simulink model "model"  (R2022a)
settings: Solver=VariableStepAuto  StartTime=0.0  StopTime=16000  RelTol=1e-3
values from neighbouring files (symbols this model uses):
  C_index = 3    [parameters.m]    (also in parameters.mat)
  C_r = 6.6    [parameters.m]    (also in parameters.mat)
  Cap_det = -1e-7    (= -1e-07)    [parameters.m]    (also in parameters.mat)
  cCap = awgn(cCap, -60)    [parameters.m]    (also in parameters.mat = [24858.4246179 23482.1280672 24461.5414582 21708.1837001 234)
  cell_count = 126    [parameters.m]    (also in parameters.mat)
  cQur = cCap / 2    [parameters.m]    (also in parameters.mat = [11880 11880 11880 11880 11880 11880 11880 11880 11880 11880)
  cTmp = 20*ones(60, 1)    [parameters.m]    (also in parameters.mat = [20 20 20 20 20 20 20 20 20 20 20 20 ... (60 elements, 60x1))
  I_CV = 1    [parameters.m]    (also in parameters.mat)
  ocv = ocv_LUT    [parameters.m]    (also in parameters.mat = [0 2.99808472822 3.29015678206 3.51449858493 3.66802196423 3)
  Q_index = 2    [parameters.m]    (also in parameters.mat)
  R_short = 33    [parameters.m]    (also in parameters.mat)
  Rp = Rp_LUT    [parameters.m]    (also in parameters.mat = [0.0013284973182 0.00132849731829 0.00133071540687 0.0013310)
  Rs = Rs_LUT    [parameters.m]    (also in parameters.mat = [0.0044622496006 0.00446224960062 0.00395928973129 0.0036572)
  soc = soc_LUT    [parameters.m]    (also in parameters.mat = [0 0.01 0.0909090909091 0.181818181818 0.272727272727 0.3636)
  tau = tau_LUT    [parameters.m]    (also in parameters.mat = [950.87194683 950.871946837 952.459545918 952.715608142 956.)
  Ts = 0.2    [parameters.m]    (also in parameters.mat)
  U_CC = 0.06    [parameters.m]    (also in parameters.mat)
  U_sought = 4.15    [parameters.m]    (also in parameters.mat)
  U_tol = 0.0000005    (= 5e-07)    [parameters.m]    (also in parameters.mat)
undefined symbols (not defined in the file or in its folder): CC_level, CC_true, CV_level, CV_true, Ts_sim
libraries: simulink x3, sharedTrackingLibrary x1, simulink_extras x1
settings Model: Creator=oscar  LastModifiedBy=oscar
settings OptimizationCC: StrengthReduction=on  PassReuseOutputArgsAs=Individual arguments  ZeroExternalMemoryAtStartup=off  ZeroInternalMemoryAtStartup=off  OptimizeBlockOrder=speed  OptimizationPriority=Speed  OptimizationCustomize=off  MultiThreadedLoops=on  EfficientTunableParamExpr=on
settings DebuggingCC: ParameterTunabilityLossMsg=error  UnconnectedInputMsg=warning  UnconnectedOutputMsg=warning  UnconnectedLineMsg=warning
settings HardwareCC: ProdBitPerPointer=32  ProdBitPerSizeT=32  ProdBitPerPtrDiffT=32  ProdLargestAtomicInteger=Long  ProdLargestAtomicFloat=Double  ProdWordSize=32  ProdHWDeviceType=ARM Compatible->ARM Cortex-M
settings SFSimCC: MATLABDynamicMemAlloc=off
settings RTWCC: SystemTargetFile=ert.tlc  GenCodeOnly=on  TemplateMakefile=ert_default_tmf  GenerateReport=on  LaunchReport=on  CodeExecutionProfiling=on  DLArmComputeVersion=19.05
settings CodeAppCC: ForceParamTrailComments=on  GenerateComments=off  IgnoreCustomStorageClasses=off  OperatorAnnotations=on  SimulinkDataObjDesc=on  SFDataObjDesc=on  InsertBlockDesc=on
settings ERTTargetCC: TargetLangStandard=C99 (ISO)  CodeReplacementLibrary=ARM Cortex-M  UtilityFuncGeneration=Shared location  GenerateSampleERTMain=on  SupportComplex=off  ERTCustomFileTemplate=example_file_process.tlc

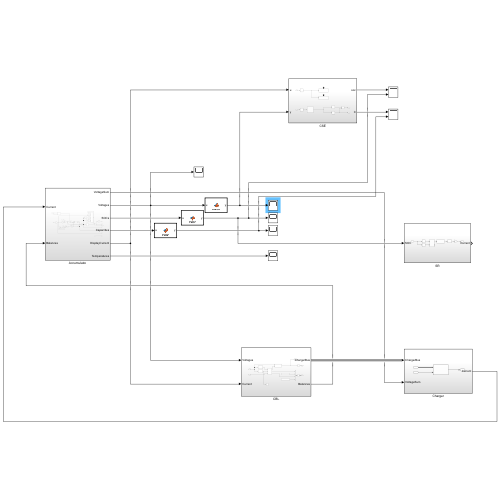
[thumbnail: Simulink's stored preview of the top-level diagram]
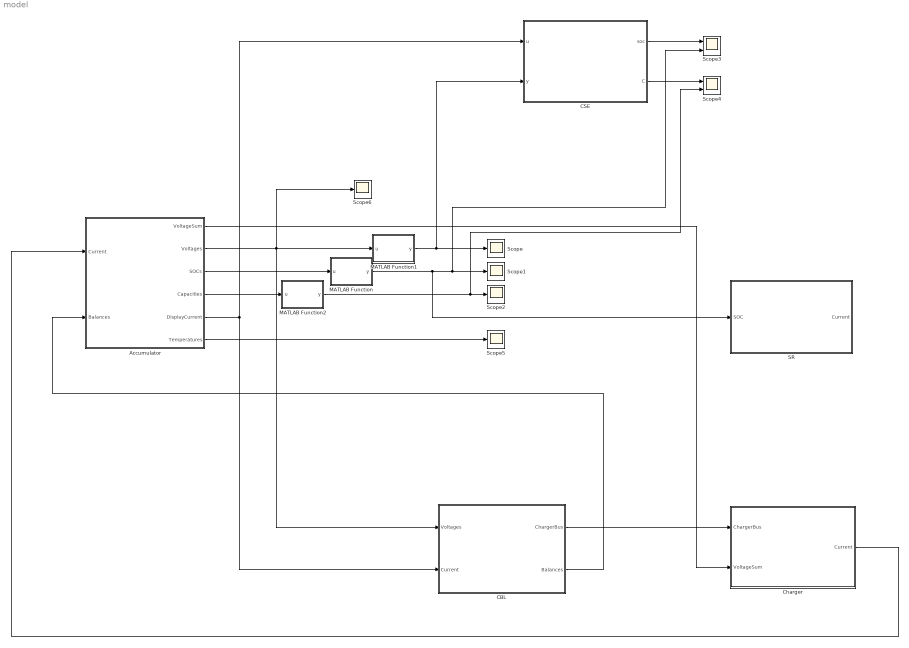
== system model ==
  Accumulator : Subsystem
  CBL : Subsystem
  CSE : Subsystem
  Charger : Subsystem
  MATLAB Function : MATLAB Function  TreatAsAtomicUnit=on
  MATLAB Function1 : MATLAB Function  TreatAsAtomicUnit=on
  MATLAB Function2 : MATLAB Function  TreatAsAtomicUnit=on
  SR : Subsystem
  Scope{,1..2,5..6} (5 alike) : Scope
  Scope3 : Scope  NumInputPorts=2
  Scope4 : Scope  NumInputPorts=2
  wires:
  Accumulator/3(SOCs) -> MATLAB Function/1(u)
  MATLAB Function/1(y) -> Scope1/1, Scope3/2, SR/1(SOC)
  Accumulator/2(Voltages) -> Scope6/1, MATLAB Function1/1(u), CBL/1(Voltages)
  MATLAB Function1/1(y) -> CSE/2(y), Scope/1
  MATLAB Function2/1(y) -> Scope4/2, Scope2/1
  Accumulator/4(Capacities) -> MATLAB Function2/1(u)
  CBL/2(Balances) -> Accumulator/2(Balances)
  CSE/1(soc) -> Scope3/1
  CSE/2(C) -> Scope4/1
  CBL/1(ChargerBus) -> Charger/1(ChargerBus)
  Accumulator/5(DisplayCurrent) -> CBL/2(Current), CSE/1(u)
  Accumulator/6(Temperatures) -> Scope5/1
  Accumulator/1(VoltageSum) -> Charger/2(VoltageSum)
  Charger/1(Current) -> Accumulator/1(Current)

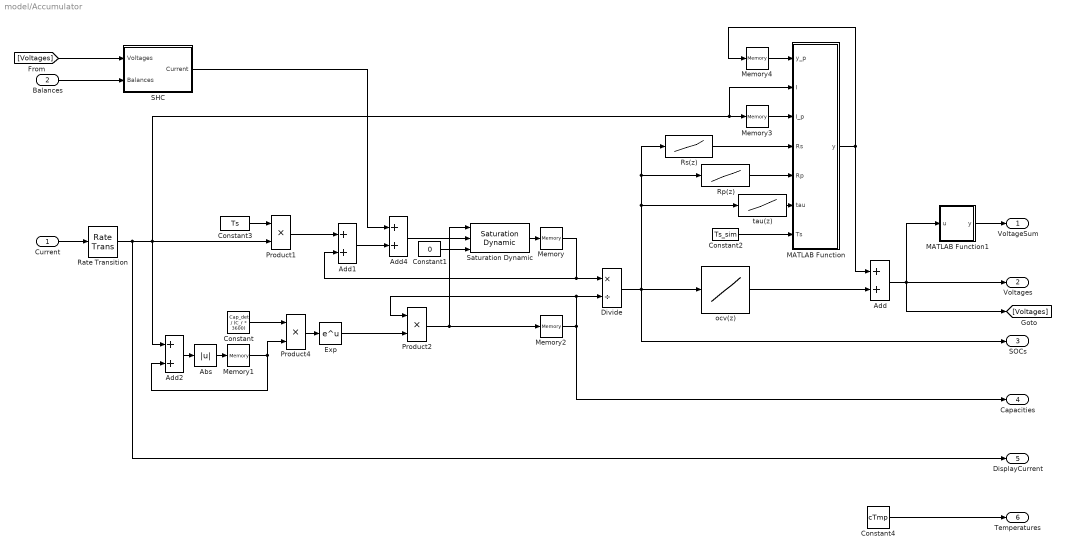
== system model/Accumulator ==
  Current : Inport
  Balances : Inport  Port=2
  Abs : Abs  SaturateOnIntegerOverflow=off
  Add{,1..2,4} (4 alike) : Sum
  Constant : Constant  Value=Cap_det / (C_r * 3600)
  Constant1 : Constant  Value=0
  Constant2 : Constant  Value=Ts_sim
  Constant3 : Constant  Value=Ts
  Constant4 : Constant  Value=cTmp
  Divide : Product  Inputs=*/
  Exp : Math
  MATLAB Function : MATLAB Function  TreatAsAtomicUnit=on
  MATLAB Function1 : MATLAB Function  TreatAsAtomicUnit=on
  Memory : Memory  InitialCondition=cQur
  Memory1 : Memory
  Memory2 : Memory  InitialCondition=cCap
  Memory3 : Memory
  Memory4 : Memory  InitialCondition=zeros(cell_count, 1)
  Product1 : Product
  Product2 : Product
  Product4 : Product
  Rate Transition : RateTransition  OutPortSampleTime=Ts
  Rp(z) : Lookup_n-D  NumberOfTableDimensions=1  BreakpointsForDimension1=soc  Table=Rp  InternalRulePriority=Speed  RndMeth=Simplest
  Rs(z) : Lookup_n-D  NumberOfTableDimensions=1  BreakpointsForDimension1=soc  Table=Rs  InternalRulePriority=Speed  RndMeth=Simplest
  SHC : Subsystem
  Saturation Dynamic : simulink/Discontinuities/Saturation Dynamic  OutMin=[]  OutMax=[]  OutDataTypeStr=Inherit: Same as second input  OutDataType=fixdt(1, 16)  OutScaling=2^-10  DoSatur=off
  ocv(z) : Lookup_n-D  NumberOfTableDimensions=1  BreakpointsForDimension1=soc  Table=ocv  InternalRulePriority=Speed  RndMeth=Simplest
  tau(z) : Lookup_n-D  NumberOfTableDimensions=1  BreakpointsForDimension1=soc  Table=tau  InternalRulePriority=Speed  RndMeth=Simplest
  VoltageSum : Outport
  Voltages : Outport  Port=2
  SOCs : Outport  Port=3
  Capacities : Outport  Port=4
  DisplayCurrent : Outport  Port=5
  Temperatures : Outport  Port=6
  wires:
  Constant/1 -> Product4/1
  Exp/1 -> Product2/2
  Product2/1 -> Saturation Dynamic/1, Memory2/1
  Memory1/1 -> Product4/2, Add2/2
  Abs/1 -> Memory1/1
  Memory/1 -> Divide/1, Add1/2
  Product4/1 -> Exp/1
  Add2/1 -> Abs/1
  Add/1 -> Voltages/1, [Voltages], MATLAB Function1/1(u)
  Saturation Dynamic/1 -> Memory/1
  Constant1/1 -> Saturation Dynamic/3
  Memory3/1 -> MATLAB Function/3(I_p)
  tau(z)/1 -> MATLAB Function/6(tau)
  Rs(z)/1 -> MATLAB Function/4(Rs)
  Rp(z)/1 -> MATLAB Function/5(Rp)
  Memory4/1 -> MATLAB Function/1(y_p)
  MATLAB Function/1(y) -> Memory4/1, Add/1
  Constant2/1 -> MATLAB Function/7(Ts)
  Current/1 -> Rate Transition/1
  Divide/1 -> ocv(z)/1, SOCs/1, tau(z)/1, Rp(z)/1, Rs(z)/1
  Memory2/1 -> Divide/2, Product2/1, Capacities/1
  ocv(z)/1 -> Add/2
  SHC/1(Current) -> Add4/1
  Balances/1 -> SHC/2(Balances)
  Add4/1 -> Saturation Dynamic/2
  [Voltages] -> SHC/1(Voltages)
  Add1/1 -> Add4/2
  Constant4/1 -> Temperatures/1
  Constant3/1 -> Product1/1
  Rate Transition/1 -> Add2/1, Product1/2, MATLAB Function/2(I), Memory3/1, DisplayCurrent/1
  Product1/1 -> Add1/1
  MATLAB Function1/1(y) -> VoltageSum/1

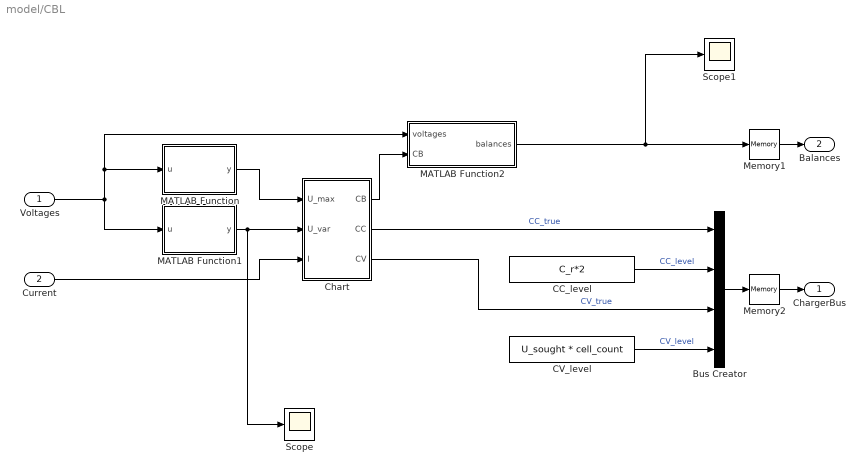
== system model/CBL ==
  Voltages : Inport
  Current : Inport  Port=2
  Bus Creator : BusCreator  Inputs=CC_true,CC_level,CV_true,CV_level
  CC_level : Constant  Value=C_r*2
  CV_level : Constant  Value=U_sought * cell_count
  Chart : Stateflow chart  TreatAsAtomicUnit=on
  MATLAB Function : MATLAB Function  TreatAsAtomicUnit=on
  MATLAB Function1 : MATLAB Function  TreatAsAtomicUnit=on
  MATLAB Function2 : MATLAB Function  TreatAsAtomicUnit=on
  Memory1 : Memory
  Memory2 : Memory
  Scope : Scope
  Scope1 : Scope
  ChargerBus : Outport
  Balances : Outport  Port=2
  wires:
  MATLAB Function/1(y) -> Chart/1(U_max)
  MATLAB Function1/1(y) -> Chart/2(U_var), Scope/1
  Voltages/1 -> MATLAB Function2/1(voltages), MATLAB Function/1(u), MATLAB Function1/1(u)
  Chart/1(CB) -> MATLAB Function2/2(CB)
  MATLAB Function2/1(balances) -> Scope1/1, Memory1/1
  Memory1/1 -> Balances/1
  Bus Creator/1 -> Memory2/1
  Current/1 -> Chart/3(I)
  CC_level/1 -> Bus Creator/2  "CC_level"
  Chart/2(CC) -> Bus Creator/1  "CC_true"
  Chart/3(CV) -> Bus Creator/3  "CV_true"
  CV_level/1 -> Bus Creator/4  "CV_level"
  Memory2/1 -> ChargerBus/1

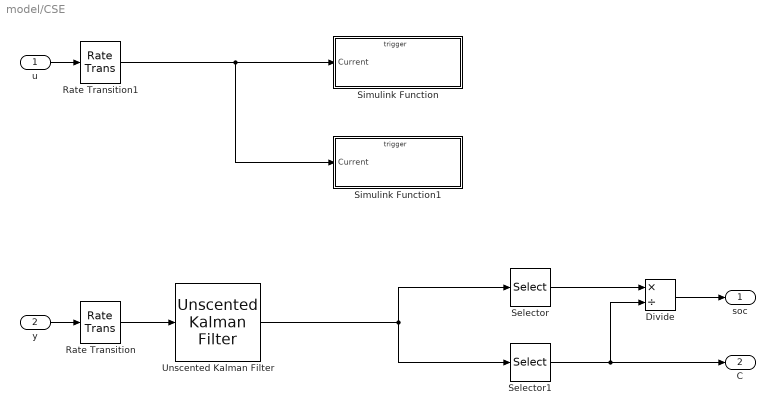
== system model/CSE ==
  u : Inport
  y : Inport  Port=2
  Divide : Product  Inputs=*/
  Rate Transition : RateTransition  OutPortSampleTime=Ts
  Rate Transition1 : RateTransition  OutPortSampleTime=Ts
  Selector : Selector  InputPortWidth=l_x  IndexOptions=Index vector (dialog)  Indices=[Q_index]  OutputSizes=1
  Selector1 : Selector  InputPortWidth=l_x  IndexOptions=Index vector (dialog)  Indices=[C_index]  OutputSizes=1
  Simulink Function : Subsystem  TreatAsAtomicUnit=on
  Simulink Function1 : Subsystem  TreatAsAtomicUnit=on
  Unscented Kalman Filter : sharedTrackingLibrary/Unscented Kalman Filter  StateTransitionFcn=S_x  HasAdditiveProcessNoise=Additive  ProcessNoise=Px0  HasTimeVaryingProcessNoise=off  HasStateTransitionFcnExtraArgument=0  InitialState=x0  InitialStateCovariance=Qx0  Alpha=1e-3  Beta=2  Kappa=0  MeasurementFcn1=M_x  HasMeasurementEnablePort1=off  HasAdditiveMeasurementNoise1=Additive  MeasurementNoise1=Rx0  HasTimeVaryingMeasurementNoise1=off  HasMeasurementFcnExtraArgument1=0  HasMeasurementWrapping1=off  MeasurementFcn2=myMeasurementFcn  HasMeasurementEnablePort2=off  HasAdditiveMeasurementNoise2=Additive  MeasurementNoise2=1  HasTimeVaryingMeasurementNoise2=off  HasMeasurementFcnExtraArgument2=0  HasMeasurementWrapping2=off  MeasurementFcn3=myMeasurementFcn  HasMeasurementEnablePort3=off  HasAdditiveMeasurementNoise3=Additive  MeasurementNoise3=1  HasTimeVaryingMeasurementNoise3=off  HasMeasurementFcnExtraArgument3=0  HasMeasurementWrapping3=off  MeasurementFcn4=myMeasurementFcn  HasMeasurementEnablePort4=off  HasAdditiveMeasurementNoise4=Additive  MeasurementNoise4=1  HasTimeVaryingMeasurementNoise4=off  HasMeasurementFcnExtraArgument4=0  HasMeasurementWrapping4=off  MeasurementFcn5=myMeasurementFcn  HasMeasurementEnablePort5=off  HasAdditiveMeasurementNoise5=Additive  MeasurementNoise5=1  HasTimeVaryingMeasurementNoise5=off  HasMeasurementFcnExtraArgument5=0  HasMeasurementWrapping5=off  EnableMultirate=off  StateTransitionFcnSampleTime=1  MeasurementFcn1SampleTime=1  MeasurementFcn2SampleTime=1  MeasurementFcn3SampleTime=1  MeasurementFcn4SampleTime=1  MeasurementFcn5SampleTime=1  UseCurrentEstimator=on  OutputStateCovariance=off  DataType=double  SampleTime=Ts  NumberOfMeasurements=1
      settings: SourceProductBaseCode=TF,AE,PW,CT,DR,ID,LP,NV,AR,RO,RR,UV,VE
  soc : Outport
  C : Outport  Port=2
  wires:
  Rate Transition/1 -> Unscented Kalman Filter/1
  Selector1/1 -> C/1, Divide/2
  Selector/1 -> Divide/1
  Divide/1 -> soc/1
  Unscented Kalman Filter/1 -> Selector1/1, Selector/1
  y/1 -> Rate Transition/1
  u/1 -> Rate Transition1/1
  Rate Transition1/1 -> Simulink Function1/1(Current), Simulink Function/1(Current)

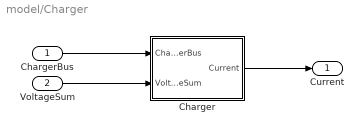
== system model/Charger ==
  ChargerBus : Inport
  VoltageSum : Inport  Port=2
  Charger : Subsystem
  Current : Outport
  wires:
  Charger/1(Current) -> Current/1
  ChargerBus/1 -> Charger/1(ChargerBus)
  VoltageSum/1 -> Charger/2(VoltageSum)

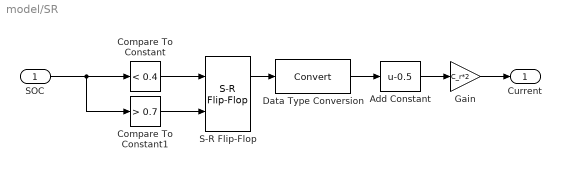
== system model/SR ==
  SOC : Inport
  Add Constant : Bias  Bias=-0.5  SaturateOnIntegerOverflow=off
  Compare To Constant : simulink/Logic and Bit Operations/Compare To Constant  relop=<  const=0.4  OutDataTypeStr=boolean
  Compare To Constant1 : simulink/Logic and Bit Operations/Compare To Constant  relop=>  const=0.7  OutDataTypeStr=boolean
  Data Type Conversion : DataTypeConversion  SaturateOnIntegerOverflow=off  RndMeth=Floor
  Gain : Gain  Gain=C_r*2
  S-R Flip-Flop : simulink_extras/Flip Flops/S-R Flip-Flop  initial_condition=0
  Current : Outport
  wires:
  Data Type Conversion/1 -> Add Constant/1
  Compare To Constant1/1 -> S-R Flip-Flop/2
  Gain/1 -> Current/1
  Add Constant/1 -> Gain/1
  S-R Flip-Flop/1 -> Data Type Conversion/1
  Compare To Constant/1 -> S-R Flip-Flop/1
  SOC/1 -> Compare To Constant1/1, Compare To Constant/1

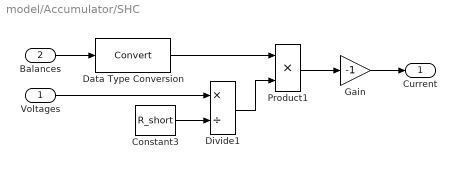
== system model/Accumulator/SHC ==
  Voltages : Inport
  Balances : Inport  Port=2
  Constant3 : Constant  Value=R_short
  Data Type Conversion : DataTypeConversion  SaturateOnIntegerOverflow=off  RndMeth=Floor
  Divide1 : Product  Inputs=*/
  Gain : Gain  Gain=-1
  Product1 : Product
  Current : Outport
  wires:
  Constant3/1 -> Divide1/2
  Data Type Conversion/1 -> Product1/1
  Divide1/1 -> Product1/2
  Balances/1 -> Data Type Conversion/1
  Product1/1 -> Gain/1
  Voltages/1 -> Divide1/1
  Gain/1 -> Current/1

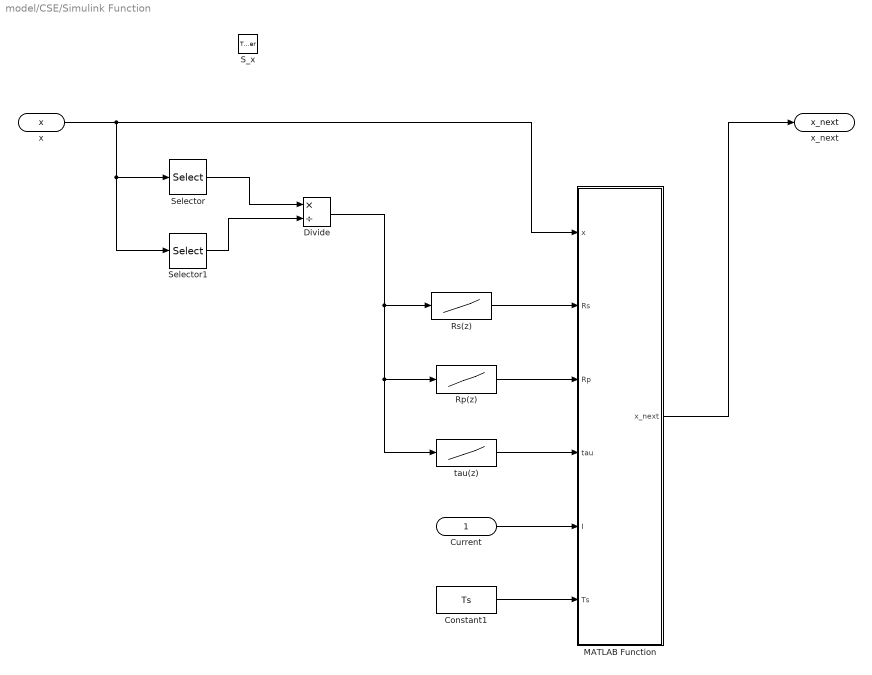
== system model/CSE/Simulink Function ==
  Current : Inport
  S_x : TriggerPort  TriggerType=function-call  IsSimulinkFunction=on  FunctionName=S_x  FunctionVisibility=scoped  VariantControl=(inherit)
  Constant1 : Constant  Value=Ts
  Divide : Product  Inputs=*/
  MATLAB Function : MATLAB Function  TreatAsAtomicUnit=on
  Rp(z) : Lookup_n-D  NumberOfTableDimensions=1  BreakpointsForDimension1=soc  Table=Rp  InternalRulePriority=Speed  RndMeth=Simplest
  Rs(z) : Lookup_n-D  NumberOfTableDimensions=1  BreakpointsForDimension1=soc  Table=Rs  InternalRulePriority=Speed  RndMeth=Simplest
  Selector : Selector  InputPortWidth=l_x  IndexOptions=Index vector (dialog)  Indices=[Q_index]  OutputSizes=1
  Selector1 : Selector  InputPortWidth=l_x  IndexOptions=Index vector (dialog)  Indices=[C_index]  OutputSizes=1
  tau(z) : Lookup_n-D  NumberOfTableDimensions=1  BreakpointsForDimension1=soc  Table=tau  InternalRulePriority=Speed  RndMeth=Simplest
  x : ArgIn  DisableCoverage=on  PortDimensions=l_x  ArgumentName=x
  x_next : ArgOut  DisableCoverage=on  PortDimensions=l_x  ArgumentName=x_next
  wires:
  Selector/1 -> Divide/1
  Rs(z)/1 -> MATLAB Function/2(Rs)
  Rp(z)/1 -> MATLAB Function/3(Rp)
  tau(z)/1 -> MATLAB Function/4(tau)
  Current/1 -> MATLAB Function/5(I)
  Constant1/1 -> MATLAB Function/6(Ts)
  MATLAB Function/1(x_next) -> x_next/1
  Selector1/1 -> Divide/2
  x/1 -> Selector1/1, Selector/1, MATLAB Function/1(x)
  Divide/1 -> Rs(z)/1, Rp(z)/1, tau(z)/1

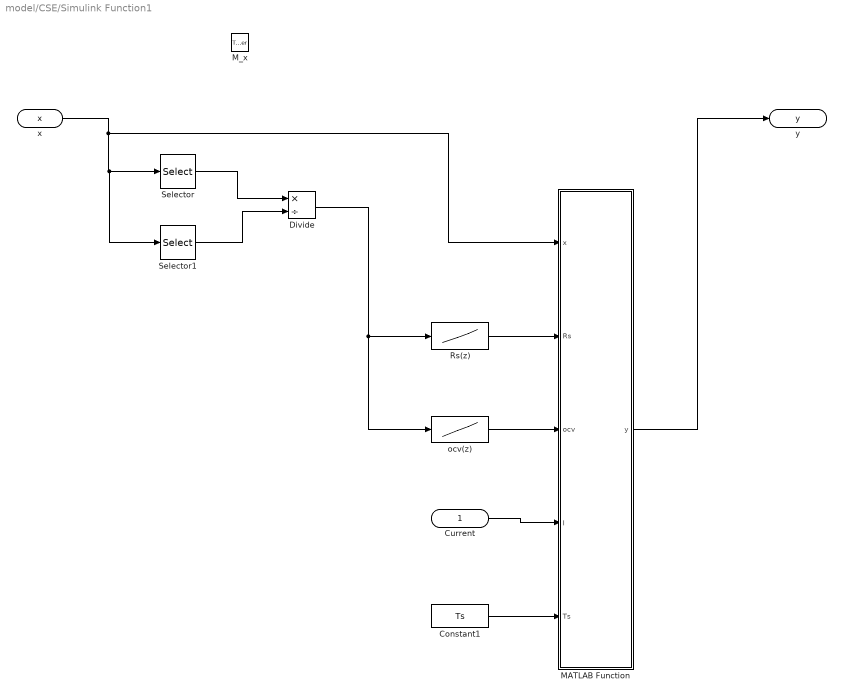
== system model/CSE/Simulink Function1 ==
  Current : Inport
  M_x : TriggerPort  TriggerType=function-call  IsSimulinkFunction=on  FunctionName=M_x  FunctionVisibility=scoped  VariantControl=(inherit)
  Constant1 : Constant  Value=Ts
  Divide : Product  Inputs=*/
  MATLAB Function : MATLAB Function  TreatAsAtomicUnit=on
  Rs(z) : Lookup_n-D  NumberOfTableDimensions=1  BreakpointsForDimension1=soc  Table=Rs  InternalRulePriority=Speed  RndMeth=Simplest
  Selector : Selector  InputPortWidth=l_x  IndexOptions=Index vector (dialog)  Indices=[Q_index]  OutputSizes=1
  Selector1 : Selector  InputPortWidth=l_x  IndexOptions=Index vector (dialog)  Indices=[C_index]  OutputSizes=1
  ocv(z) : Lookup_n-D  NumberOfTableDimensions=1  BreakpointsForDimension1=soc  Table=ocv  InternalRulePriority=Speed  RndMeth=Simplest
  x : ArgIn  DisableCoverage=on  PortDimensions=l_x  ArgumentName=x
  y : ArgOut  DisableCoverage=on  ArgumentName=y
  wires:
  Rs(z)/1 -> MATLAB Function/2(Rs)
  Current/1 -> MATLAB Function/4(I)
  MATLAB Function/1(y) -> y/1
  ocv(z)/1 -> MATLAB Function/3(ocv)
  Selector/1 -> Divide/1
  x/1 -> Selector1/1, Selector/1, MATLAB Function/1(x)
  Selector1/1 -> Divide/2
  Divide/1 -> ocv(z)/1, Rs(z)/1
  Constant1/1 -> MATLAB Function/5(Ts)

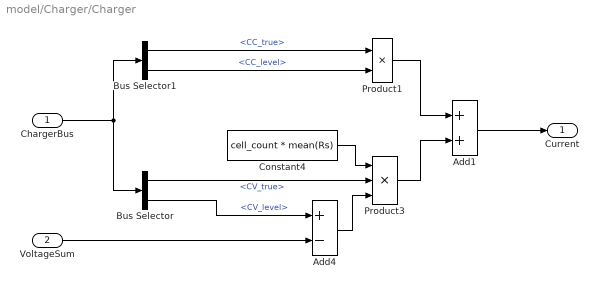
== system model/Charger/Charger ==
  ChargerBus : Inport
  VoltageSum : Inport  Port=2
  Add1 : Sum
  Add4 : Sum  Inputs=+-
  Bus Selector : BusSelector  OutputSignals=CV_true,CV_level
  Bus Selector1 : BusSelector  OutputSignals=CC_true,CC_level
  Constant4 : Constant  Value=cell_count * mean(Rs)
  Product1 : Product
  Product3 : Product  Inputs=3
  Current : Outport
  wires:
  Bus Selector/1 -> Product3/2  "<CV_true>"
  Add4/1 -> Product3/3
  VoltageSum/1 -> Add4/2
  Bus Selector/2 -> Add4/1  "<CV_level>"
  Constant4/1 -> Product3/1
  ChargerBus/1 -> Bus Selector1/1, Bus Selector/1
  Bus Selector1/1 -> Product1/1  "<CC_true>"
  Bus Selector1/2 -> Product1/2  "<CC_level>"
  Product1/1 -> Add1/1
  Product3/1 -> Add1/2
  Add1/1 -> Current/1

== matlab function model/CSE/Simulink Function1/MATLAB Function ==
  data: x input; y output; Rs input; ocv input; I input; Ts input
function y = h(x, Rs, ocv, I, Ts)

y = ocv + I * Rs + x(1);

end

== matlab function model/Accumulator/MATLAB Function ==
  data: y_p input; I input; y output; I_p input; Rs input; Rp input; tau input; Ts input
function y = mTustin(y_p, I, I_p, Rs, Rp, tau, Ts)

a = Rs.*tau;
b = Rs + Rp;
c = tau;
d = ones(length(tau), 1);

a_ = Ts*b + 2*a;
b_ = Ts*b - 2*a;
c_ = Ts*d + 2*c;
d_ = Ts*d - 2*c;

y = (a_ .*I + b_ .* I_p - d_ .* y_p) ./ c_;

== matlab function model/Accumulator/MATLAB Function1 ==
  data: u input; y output
function y = sum(u)

y = sum(u);

== matlab function model/MATLAB Function ==
  data: u input; y output
function y = mean(u)

y = mean(u);

== matlab function model/MATLAB Function1 ==
  data: u input; y output
function y = mean(u)

y = mean(u);

== matlab function model/MATLAB Function2 ==
  data: u input; y output
function y = mean(u)

y = mean(u);

== stateflow chart model/CBL/Chart ==
  state Entry_
    CC = 0;
    CV = 0;
    CB = 0;
  state CC_state_
    CC = 1;
    CV = 0;
    CB = 0;
  state CV_state_
    CC = 0;
    CV = 1;
    CB = 0;
  state CB_state_
    CC = 0;
    CV = 0;
    CB = 1;
  (default) -> Entry_
  Entry_ -> CC_state_ [order 1] : [U_max < (U_sought - U_CC)]
  CC_state_ -> CV_state_ : [U_max > (U_sought - U_CC)]
  Entry_ -> CB_state_ [order 2] : [U_var > U_tol]
  CB_state_ -> Entry_ [order 1] : [U_var < U_tol]
  CB_state_ -> CC_state_ [order 2] : [U_max < (U_sought - U_CC)]
  CV_state_ -> CB_state_ : [I^2 < I_CV^2]
  data: U_max input; U_var input; CB output; CC output; CV output; U_CC parameter; U_tol parameter double; U_sought parameter; I_CV parameter; I input

== matlab function model/CBL/MATLAB Function ==
  data: u input; y output
function y = max(u)

y = max(u);

== matlab function model/CBL/MATLAB Function1 ==
  data: u input; y output
function y = var(u)

y = var(u);

== matlab function model/CBL/MATLAB Function2 ==
  data: voltages input; balances output; CB input
function balances = strategy(voltages, CB)
balances = voltages*0;

if CB
    [~, I] = sort(voltages, 'descend');
    for k = 1:36
        balances(I(k)) = 1;
    end
end

== matlab function model/CSE/Simulink Function/MATLAB Function ==
  data: x input; x_next output; Rs input; Rp input; tau input; I input; Ts input
function x_next = f(x, Rs, Rp, tau, I, Ts)
x_next = zeros(3, 1);

x_next(1) = exp(-Ts / tau) * x(1) + I * (1 - exp(-Ts / tau)) * Rp;
x_next(2) = x(2) + I * Ts;
x_next(3) = x(3);
end
